simulink model "Noh_Nofusion"  (R2020b)
settings: Solver=FixedStepAuto  StartTime=0.0  StopTime=Inf  FixedStep=0.01  RelTol=1e-3
PostLoadFcn:
  | if any(exist('dsrtsu_mdlpostloadfcn', 'file') ~= 0), dsrtsu_mdlpostloadfcn('Execute', bdroot); end
InitFcn:
  | , if any(exist('rtifpga_mdlclblib', 'file') ~= 0), rtifpga_mdlclblib('Init', bdroot); end,
  | , if any(exist('dsmpb_private', 'file') ~= 0), dsmpb_private('dsmpb_mdlclblib', 'Init', bdroot); end,
undefined symbols (not defined in the file): ACC_TimeGap_DecSetSwt, ACC_TimeGap_IncSetSwt, AccelPedalPosn, AccelPedalPosnVldty, AccelPedlPosnDiagc, AccPedalOverride, ACU_ShiftInProgress, ADAS_Posn_CurLane, AESSwtReq, ALC_SwtReq, BrkPedalSts, CC_ACC_CANCEL_OFFSwt, CC_ACC_CRUISE_OFFSwt, CC_ACC_DecSetSpd_SetSwt, CC_ACC_IncSetSpd_ResuSwt, CC_ACCSwtErr, CharSpd_ms, CSA_NODE, CURRENT_GEAR, CurrentGearValid, DiscIntNeverNeededParam, DrvDoorSts, DrvSBR, DrvTrqReqOvld, ECMACCInterface, ECMRespACC, ELKSwtReq, EngLimpHomeSts, EngSpd, EngState, EngState_PHEV, EngTrqMaxActSpd, EngTrqMinAct, EPS_DrvInpTrqVal_HighReslolution, EPS_FailSts, EPS_LKATorqOvrlDlvd, EPS_LKATorqOvrlDlvdVld, EPS_LKATrqOvlDlvdSts, EPS_SteerMod, EPS_TrqSnsrSts, EQ4_APPINFO, EQ4_LA_ELEM, EQ4_LA_HDR, EQ4_LAP_ELEM, EQ4_LAP_HDR, EQ4_LH_ELEM, EQ4_LH_HDR, EQ4_LRE_ELEM, EQ4_LRE_HDR, ESS_PedSwtReq, ESS_VehSwtReq, FFogLmpSts_F_Pbox, FLWheelDriveDirection, FLWheelSpd, FrntWiprSwtSts, FrntWshrSwtSts, FRWheelDriveDirection, FRWheelSpd, HazardLmpSwtSts, HCU_AccelPedalPosn_Diag ... (+153)
libraries: simulink x132, dsmpblib x27
(part 6 of 14)

== system Noh_Nofusion/LPV/HAP_Pack ==
  In1 : Inport
  Bus Assignment2 : BusAssignment  AssignedSignals=USS_FrontSys_Status,USS_FLCNear_Obj_Confidence,USS_FLCNear_Obj_Pos_X,USS_FLCNear_Obj_Pos_Y,USS_FLMNear_Obj_Confidence,USS_FLMNear_Obj_Pos_X,USS_FLMNear_Obj_Pos_Y,USS_FRMNear_Obj_Confidence,USS_FRMNear_Obj_Pos_X,USS_FRMNear_Obj_Pos_Y,USS_FRCNear_Obj_Confidence,USS_FRCNear_Obj_Pos_X,USS_FRCNear_Obj_Pos_Y,APS_WorkSts,DVRWorkSts
  Bus Selector18 : BusSelector  OutputSignals=HAP_NODE.HAP_FD6_MSG.USS_FrontSys_Status,HAP_NODE.HAP_FD6_MSG.USS_FLCNear_Obj_Confidence,HAP_NODE.HAP_FD6_MSG.USS_FLCNear_Obj_Pos_X,HAP_NODE.HAP_FD6_MSG.USS_FLCNear_Obj_Pos_Y,HAP_NODE.HAP_FD6_MSG.USS_FLMNear_Obj_Confidence,HAP_NODE.HAP_FD6_MSG.USS_FLMNear_Obj_Pos_X,HAP_NODE.HAP_FD6_MSG.USS_FLMNear_Obj_Pos_Y,HAP_NODE.HAP_FD6_MSG.USS_FRMNear_Obj_Confidence,HAP_NODE.HAP_FD6_MSG.USS_FRMNear_Obj_Pos_X,HAP_NODE.HAP_FD6_MSG.USS_FRMNear_Obj_Pos_Y,HAP_NODE.HAP_FD6_MSG.USS_FRCNear_Obj_Confidence,HAP_NODE.HAP_FD6_MSG.USS_FRCNear_Obj_Pos_X,HAP_NODE.HAP_FD6_MSG.USS_FRCNear_Obj_Pos_Y,HAP_NODE.HAP_FD1_MSG.APS_WorkSts,HAP_NODE.HAP_FD2_MSG.DVRWorkSts
  Constant3 : Constant  Value=0  OutDataTypeStr=Bus: VCAN_HAP_MSG_BUS
  VSM_VCAN_HAP : Outport
  wires:
  Bus Assignment2/1 -> VSM_VCAN_HAP/1
  Bus Selector18/15 -> Bus Assignment2/16  "<DVRWorkSts>"
  Bus Selector18/14 -> Bus Assignment2/15  "<APS_WorkSts>"
  Bus Selector18/13 -> Bus Assignment2/14  "<USS_FRCNear_Obj_Pos_Y>"
  Bus Selector18/12 -> Bus Assignment2/13  "<USS_FRCNear_Obj_Pos_X>"
  Bus Selector18/11 -> Bus Assignment2/12  "<USS_FRCNear_Obj_Confidence>"
  Bus Selector18/10 -> Bus Assignment2/11  "<USS_FRMNear_Obj_Pos_Y>"
  Bus Selector18/9 -> Bus Assignment2/10  "<USS_FRMNear_Obj_Pos_X>"
  Bus Selector18/8 -> Bus Assignment2/9  "<USS_FRMNear_Obj_Confidence>"
  Bus Selector18/7 -> Bus Assignment2/8  "<USS_FLMNear_Obj_Pos_Y>"
  Bus Selector18/6 -> Bus Assignment2/7  "<USS_FLMNear_Obj_Pos_X>"
  Bus Selector18/5 -> Bus Assignment2/6  "<USS_FLMNear_Obj_Confidence>"
  Bus Selector18/4 -> Bus Assignment2/5  "<USS_FLCNear_Obj_Pos_Y>"
  Bus Selector18/3 -> Bus Assignment2/4  "<USS_FLCNear_Obj_Pos_X>"
  Bus Selector18/2 -> Bus Assignment2/3  "<USS_FLCNear_Obj_Confidence>"
  Bus Selector18/1 -> Bus Assignment2/2  "<USS_FrontSys_Status>"
  Constant3/1 -> Bus Assignment2/1
  In1/1 -> Bus Selector18/1

== system Noh_Nofusion/LPV/HUT_Pack ==
  In1 : Inport
  Bus Assignment1 : BusAssignment  AssignedSignals=CR_BrkgReq
  Bus Assignment2 : BusAssignment  AssignedSignals=IFC_SnvtySet,LKASwtReq,LCKSwtReq,ELKSwtReq,ESS_PedSwtReq,ESS_VehSwtReq,LDWSwtReq,TSRSwtReq,TSRWarnSwtReq,ICA_HandsOffSwtReq,ISLSwtReq,TSR_SnvtySet,LSSWarnFormSwtReq,LSSSwtReq,IntelligentEvaSwtReq,AESSwtReq,HWA_SwtReq,HWA_SnvtySet,ALC_SwtReq
  Bus Selector16 : BusSelector  OutputSignals=HUT_NODE.HUT_FD1_MSG.IFC_SnvtySet,HUT_NODE.HUT_FD1_MSG.LKASwtReq,HUT_NODE.HUT_FD1_MSG.LCKSwtReq,HUT_NODE.HUT_FD1_MSG.ELKSwtReq,HUT_NODE.HUT_FD1_MSG.ESS_PedSwtReq,HUT_NODE.HUT_FD1_MSG.ESS_VehSwtReq,HUT_NODE.HUT_FD1_MSG.LDWSwtReq,HUT_NODE.HUT_FD1_MSG.TSRSwtReq,HUT_NODE.HUT_FD1_MSG.TSRWarnSwtReq,HUT_NODE.HUT_FD1_MSG.ICA_HandsOffSwtReq,HUT_NODE.HUT_FD1_MSG.ISLSwtReq,HUT_NODE.HUT_FD1_MSG.TSR_SnvtySet,HUT_NODE.HUT_FD1_MSG.LSSWarnFormSwtReq,HUT_NODE.HUT_FD1_MSG.LSSSwtReq,HUT_NODE.HUT_FD1_MSG.IntelligentEvaSwtReq,HUT_NODE.HUT_FD1_MSG.AESSwtReq,HUT_NODE.HUT_FD1_MSG.HWA_SwtReq,HUT_NODE.HUT_FD1_MSG.HWA_SnvtySet,HUT_NODE.HUT_FD1_MSG.ALC_SwtReq,CR_NODE.CR_FD1_MSG.CR_BrkgReq
  Constant1 : Constant  Value=0  OutDataTypeStr=Bus: VCAN_CR_MSG_BUS
  Constant3 : Constant  Value=0  OutDataTypeStr=Bus: VCAN_HUT_MSG_BUS
  VSM_VCAN_HUT : Outport
  VSM_VCAN_CR : Outport  Port=2
  wires:
  Bus Assignment1/1 -> VSM_VCAN_CR/1
  Bus Selector16/20 -> Bus Assignment1/2  "<CR_BrkgReq>"
  Constant1/1 -> Bus Assignment1/1
  Bus Assignment2/1 -> VSM_VCAN_HUT/1
  Bus Selector16/19 -> Bus Assignment2/20  "<ALC_SwtReq>"
  Bus Selector16/18 -> Bus Assignment2/19  "<HWA_SnvtySet>"
  Bus Selector16/17 -> Bus Assignment2/18  "<HWA_SwtReq>"
  Bus Selector16/16 -> Bus Assignment2/17  "<AESSwtReq>"
  Bus Selector16/15 -> Bus Assignment2/16  "<IntelligentEvaSwtReq>"
  Bus Selector16/14 -> Bus Assignment2/15  "<LSSSwtReq>"
  Bus Selector16/13 -> Bus Assignment2/14  "<LSSWarnFormSwtReq>"
  Bus Selector16/12 -> Bus Assignment2/13  "<TSR_SnvtySet>"
  Bus Selector16/11 -> Bus Assignment2/12  "<ISLSwtReq>"
  Bus Selector16/10 -> Bus Assignment2/11  "<ICA_HandsOffSwtReq>"
  Bus Selector16/9 -> Bus Assignment2/10  "<TSRWarnSwtReq>"
  Bus Selector16/8 -> Bus Assignment2/9  "<TSRSwtReq>"
  Bus Selector16/7 -> Bus Assignment2/8  "<LDWSwtReq>"
  Bus Selector16/6 -> Bus Assignment2/7  "<ESS_VehSwtReq>"
  Bus Selector16/5 -> Bus Assignment2/6  "<ESS_PedSwtReq>"
  Bus Selector16/4 -> Bus Assignment2/5  "<ELKSwtReq>"
  Bus Selector16/3 -> Bus Assignment2/4  "<LCKSwtReq>"
  Bus Selector16/2 -> Bus Assignment2/3  "<LKASwtReq>"
  Bus Selector16/1 -> Bus Assignment2/2  "<IFC_SnvtySet>"
  Constant3/1 -> Bus Assignment2/1
  In1/1 -> Bus Selector16/1

== system Noh_Nofusion/LPV/Subsystem ==
  In1 : Inport
  Bus Assignment2 : BusAssignment  AssignedSignals=ACAmbTemp
  Bus Selector11 : BusSelector  OutputSignals=AC_NEDE.AC2_MSG.ACAmbTemp
  Constant3 : Constant  Value=0  OutDataTypeStr=Bus: VCAN_AC_MSG_BUS
  <ACAmbTemp> : Outport
  wires:
  Bus Assignment2/1 -> <ACAmbTemp>/1
  Constant3/1 -> Bus Assignment2/1
  Bus Selector11/1 -> Bus Assignment2/2  "<ACAmbTemp>"
  In1/1 -> Bus Selector11/1

== system Noh_Nofusion/LPV/Subsystem1 ==
  In1 : Inport
  Bus Assignment2 : BusAssignment  AssignedSignals=IP_VehSpdUnit
  Bus Selector15 : BusSelector  OutputSignals=IP_NODE.IP2_MSG.IP_VehSpdUnit
  Constant3 : Constant  Value=0  OutDataTypeStr=Bus: VCAN_IP_MSG_BUS
  <IP_VehSpdUnit> : Outport
  wires:
  Bus Assignment2/1 -> <IP_VehSpdUnit>/1
  Bus Selector15/1 -> Bus Assignment2/2  "<IP_VehSpdUnit>"
  Constant3/1 -> Bus Assignment2/1
  In1/1 -> Bus Selector15/1

== system Noh_Nofusion/LPV/Subsystem2 ==
  In1 : Inport
  Bus Assignment2 : BusAssignment  AssignedSignals=HighBeamSts_HC
  Bus Selector17 : BusSelector  OutputSignals=HC_NODE.HC1_MSG.HighBeamSts_HC
  Constant3 : Constant  Value=0  OutDataTypeStr=Bus: VCAN_HC_MSG_BUS
  <HighBeamSts_HC> : Outport
  wires:
  Bus Assignment2/1 -> <HighBeamSts_HC>/1
  Bus Selector17/1 -> Bus Assignment2/2  "<HighBeamSts_HC>"
  Constant3/1 -> Bus Assignment2/1
  In1/1 -> Bus Selector17/1

== system Noh_Nofusion/LPV/Subsystem3 ==
  In1 : Inport
  Bus Assignment2 : BusAssignment  AssignedSignals=HoodSts_F_Pbox,FFogLmpSts_F_Pbox,RFogLmpSts_R_Pbox,LowBeamSts_F_Pbox
  Bus Selector12 : BusSelector  OutputSignals=PBOX_NODE.F_PBOX1_MSG.HoodSts_F_Pbox,PBOX_NODE.F_PBOX1_MSG.FFogLmpSts_F_Pbox,PBOX_NODE.R_PBOX1_MSG.RFogLmpSts_R_Pbox,PBOX_NODE.F_PBOX1_MSG.LowBeamSts_F_Pbox
  Constant3 : Constant  Value=0  OutDataTypeStr=Bus: VCAN_PBOX_MSG_BUS
  VSM_VCAN_PBOX : Outport
  wires:
  Bus Selector12/1 -> Bus Assignment2/2  "<HoodSts_F_Pbox>"
  Bus Selector12/2 -> Bus Assignment2/3  "<FFogLmpSts_F_Pbox>"
  Bus Selector12/3 -> Bus Assignment2/4  "<RFogLmpSts_R_Pbox>"
  Bus Selector12/4 -> Bus Assignment2/5  "<LowBeamSts_F_Pbox>"
  Constant3/1 -> Bus Assignment2/1
  In1/1 -> Bus Selector12/1
  Bus Assignment2/1 -> VSM_VCAN_PBOX/1

== system Noh_Nofusion/LPV/Subsystem4 ==
  In1 : Inport
  Bus Assignment4 : BusAssignment  AssignedSignals=HCU_BrkPedalSts,HCU_AccelPedalPosn_Diag,HCU_ACCInterface,HCU_PowertrainSts,ACU_ShiftInProgress,HCU_DrvMod,HCU_PTDrvMod,DrvTrqReqOvld,HCU_GearSts
  Bus Selector11 : BusSelector  OutputSignals=HCU_NODE.HCU_FD1_MSG.HCU_BrkPedalSts,HCU_NODE.HCU_FD1_MSG.HCU_AccelPedalPosn_Diag,HCU_NODE.HCU_FD1_MSG.HCU_ACCInterface,HCU_NODE.HCU_FD1_MSG.HCU_PowertrainSts,HCU_NODE.HCU_FD1_MSG.ACU_ShiftInProgress,HCU_NODE.HCU_FD3_MSG.HCU_DrvMod,HCU_NODE.HCU_FD3_MSG.HCU_PTDrvMod,HCU_NODE.HCU_FD3_MSG.DrvTrqReqOvld,HCU_NODE.HCU_FD3_MSG.HCU_GearSts
  Constant4 : Constant  Value=0  OutDataTypeStr=Bus: VCAN_HCU_MSG_BUS
  Out1 : Outport
  wires:
  In1/1 -> Bus Selector11/1
  Bus Selector11/9 -> Bus Assignment4/10  "<HCU_GearSts>"
  Bus Selector11/7 -> Bus Assignment4/8  "<HCU_PTDrvMod>"
  Bus Selector11/3 -> Bus Assignment4/4  "<HCU_ACCInterface>"
  Bus Assignment4/1 -> Out1/1
  Bus Selector11/2 -> Bus Assignment4/3  "<HCU_AccelPedalPosn_Diag>"
  Bus Selector11/5 -> Bus Assignment4/6  "<ACU_ShiftInProgress>"
  Bus Selector11/8 -> Bus Assignment4/9  "<DrvTrqReqOvld>"
  Bus Selector11/1 -> Bus Assignment4/2  "<HCU_BrkPedalSts>"
  Constant4/1 -> Bus Assignment4/1
  Bus Selector11/6 -> Bus Assignment4/7  "<HCU_DrvMod>"
  Bus Selector11/4 -> Bus Assignment4/5  "<HCU_PowertrainSts>"

== system Noh_Nofusion/LPV/Subsystem5 ==
  TOS_P0_TARGET_LINE : Inport  OutDataTypeStr=Bus: TOS_P0_TARGET_LINE_BUS  PortDimensions=1  BusOutputAsStruct=on
  VSM_HMI : Inport  Port=2  OutDataTypeStr=Bus: VSM_HMI_BUS  PortDimensions=1  BusOutputAsStruct=on
  VSM_ReqMRC : Inport  Port=3  OutDataTypeStr=uint8
  vxvRefMs : Inport  Port=4  OutDataTypeStr=single  PortDimensions=1  BusOutputAsStruct=on
  kapTraj : Inport  Port=5  OutDataTypeStr=single  PortDimensions=1  BusOutputAsStruct=on
  PLAN_ALC_DECS : Inport  Port=6  OutDataTypeStr=Bus: PLAN_ALC_DECS_BUS  PortDimensions=1  BusOutputAsStruct=on
  RFM_ROAD : Inport  Port=7  OutDataTypeStr=Bus: RFM_ROAD_BUS  PortDimensions=1  BusOutputAsStruct=on
  RFM_UpdateCnt : Inport  Port=8  OutDataTypeStr=uint32  PortDimensions=1  BusOutputAsStruct=on
  RFM_BRANCH_LANE : Inport  Port=9  OutDataTypeStr=Bus: RFM_LANE_BUS  PortDimensions=1  BusOutputAsStruct=on
  RFM_LEFT_LANE : Inport  Port=10  OutDataTypeStr=Bus: RFM_LANE_BUS  PortDimensions=1  BusOutputAsStruct=on
  RFM_CURRENT_LANE : Inport  Port=11  OutDataTypeStr=Bus: RFM_LANE_BUS  PortDimensions=1  BusOutputAsStruct=on
  RFM_RIGHT_LANE : Inport  Port=12  OutDataTypeStr=Bus: RFM_LANE_BUS  PortDimensions=1  BusOutputAsStruct=on
  RFM_INTERSEC_ALERT : Inport  Port=13  OutDataTypeStr=Bus: RFM_INTERSEC_ALERT_BUS  PortDimensions=1  BusOutputAsStruct=on
  RFM_BRANCH : Inport  Port=14  OutDataTypeStr=Bus: RFM_BRANCH_BUS  PortDimensions=1  BusOutputAsStruct=on
  RFM_REC_LANES : Inport  Port=15  OutDataTypeStr=Bus: RFM_REC_LANES_BUS  PortDimensions=1  BusOutputAsStruct=on
  RFM_LINE_L1 : Inport  Port=16  OutDataTypeStr=Bus: RFM_LINE_BUS  PortDimensions=1  BusOutputAsStruct=on
  RFM_LINE_R1 : Inport  Port=17  OutDataTypeStr=Bus: RFM_LINE_BUS  PortDimensions=1  BusOutputAsStruct=on
  RFM_LINE_L2 : Inport  Port=18  OutDataTypeStr=Bus: RFM_LINE_BUS  PortDimensions=1  BusOutputAsStruct=on
  RFM_LINE_R2 : Inport  Port=19  OutDataTypeStr=Bus: RFM_LINE_BUS  PortDimensions=1  BusOutputAsStruct=on
  RFM_LINE_L3 : Inport  Port=20  OutDataTypeStr=Bus: RFM_LINE_BUS  PortDimensions=1  BusOutputAsStruct=on
  RFM_LINE_R3 : Inport  Port=21  OutDataTypeStr=Bus: RFM_LINE_BUS  PortDimensions=1  BusOutputAsStruct=on
  RFM_LINE_CL : Inport  Port=22  OutDataTypeStr=Bus: RFM_LINE_BUS  PortDimensions=1  BusOutputAsStruct=on
  RFM_LINE_LB : Inport  Port=23  OutDataTypeStr=Bus: RFM_LINE_BUS  PortDimensions=1  BusOutputAsStruct=on
  RFM_LINE_RB : Inport  Port=24  OutDataTypeStr=Bus: RFM_LINE_BUS  PortDimensions=1  BusOutputAsStruct=on
  RFM_LINE_PRED : Inport  Port=25  OutDataTypeStr=Bus: RFM_LINE_BUS  PortDimensions=1  BusOutputAsStruct=on
  RFM_LINEF_LB : Inport  Port=26  OutDataTypeStr=Bus: RFM_LINE_BUS  PortDimensions=1  BusOutputAsStruct=on
  RFM_LINEF_RB : Inport  Port=27  OutDataTypeStr=Bus: RFM_LINE_BUS  PortDimensions=1  BusOutputAsStruct=on
  RFM_LINE_ENTRY_CL : Inport  Port=28  OutDataTypeStr=Bus: RFM_LINE_BUS  PortDimensions=1  BusOutputAsStruct=on
  RFM_LINE_EXIT_CL : Inport  Port=29  OutDataTypeStr=Bus: RFM_LINE_BUS  PortDimensions=1  BusOutputAsStruct=on
  EQ4_LH_HDR : Inport  Port=30  OutDataTypeStr=Bus: EQ4_LH_HDR_BUS  PortDimensions=1  BusOutputAsStruct=on
  EQ4_LH_ELEM : Inport  Port=31  OutDataTypeStr=Bus: EQ4_LH_ELEM_BUS  PortDimensions=1  BusOutputAsStruct=on
  EQ4_LH_ELEM1 : Inport  Port=32  OutDataTypeStr=Bus: EQ4_LH_ELEM_BUS  PortDimensions=1  BusOutputAsStruct=on
  EQ4_LA_HDR : Inport  Port=33  OutDataTypeStr=Bus: EQ4_LA_HDR_BUS  PortDimensions=1  BusOutputAsStruct=on
  EQ4_LA_ELEM : Inport  Port=34  OutDataTypeStr=Bus: EQ4_LA_ELEM_BUS  PortDimensions=1  BusOutputAsStruct=on
  EQ4_LA_ELEM1 : Inport  Port=35  OutDataTypeStr=Bus: EQ4_LA_ELEM_BUS  PortDimensions=1  BusOutputAsStruct=on
  EQ4_LA_ELEM2 : Inport  Port=36  OutDataTypeStr=Bus: EQ4_LA_ELEM_BUS  PortDimensions=1  BusOutputAsStruct=on
  EQ4_LA_ELEM3 : Inport  Port=37  OutDataTypeStr=Bus: EQ4_LA_ELEM_BUS  PortDimensions=1  BusOutputAsStruct=on
  EQ4_LRE_HDR : Inport  Port=38  OutDataTypeStr=Bus: EQ4_LRE_HDR_BUS  PortDimensions=1  BusOutputAsStruct=on
  EQ4_LRE_ELEM : Inport  Port=39  OutDataTypeStr=Bus: EQ4_LRE_ELEM_BUS  PortDimensions=1  BusOutputAsStruct=on
  EQ4_LRE_ELEM1 : Inport  Port=40  OutDataTypeStr=Bus: EQ4_LRE_ELEM_BUS  PortDimensions=1  BusOutputAsStruct=on
  RFM_TSR : Inport  Port=41  OutDataTypeStr=Bus: RFM_TSR_BUS  PortDimensions=1  BusOutputAsStruct=on
  Bus Assignment1 : BusAssignment  AssignedSignals=EQ4_LH_HDR,EQ4_LH_ELEM
  Bus Assignment2 : BusAssignment  AssignedSignals=EQ4_LRE_HDR,EQ4_LRE_ELEM
  Bus Assignment3 : BusAssignment  AssignedSignals=EQ4_LA_HDR,EQ4_LA_ELEM
  Constant1 : Constant  Value=0  OutDataTypeStr=Bus: EQ4_LA_BUS
  Constant2 : Constant  Value=0  OutDataTypeStr=Bus: EQ4_LH_BUS
  Constant3 : Constant  Value=0  OutDataTypeStr=Bus: EQ4_LRE_BUS
  For Each Subsystem1 : Subsystem  TreatAsAtomicUnit=on
  For Each Subsystem2 : Subsystem  TreatAsAtomicUnit=on
  For Each Subsystem3 : Subsystem  TreatAsAtomicUnit=on
  LSM : ModelReference  ModelNameDialog=PubIfDecisionLSM_MDL.slx  SimulationMode=Normal  ModelReferenceVersion=1.510
  Matrix Concatenate : Concatenate  Mode=Multidimensional array
  Matrix Concatenate1 : Concatenate  NumInputs=4  Mode=Multidimensional array
  Matrix Concatenate2 : Concatenate  Mode=Multidimensional array
  Terminator : Terminator
  LSM_TJA_ICA : Outport  OutDataTypeStr=Bus: LSM_TJA_ICA_BUS  PortDimensions=1  BusOutputAsStruct=on
  LSM_LCK : Outport  Port=2  OutDataTypeStr=Bus: LSM_LCK_BUS  PortDimensions=1  BusOutputAsStruct=on
  LSM_HWA : Outport  Port=3  OutDataTypeStr=Bus: LSM_HWA_BUS  PortDimensions=1  BusOutputAsStruct=on
  LSM_ESS : Outport  Port=4  OutDataTypeStr=Bus: LSM_ESS_BUS  PortDimensions=1  BusOutputAsStruct=on
  LSM_UpdateCnt : Outport  Port=5  OutDataTypeStr=uint32  PortDimensions=1  BusOutputAsStruct=on
  LSM_PilotTurnSwSts : Outport  Port=6  OutDataTypeStr=uint8  PortDimensions=1  BusOutputAsStruct=on
  LSM_PilotSts : Outport  Port=7  OutDataTypeStr=uint8  PortDimensions=1  BusOutputAsStruct=on
  LSM_PilotNohExitDist : Outport  Port=8  OutDataTypeStr=uint16  PortDimensions=1  BusOutputAsStruct=on
  LSM_PilotSPLDist : Outport  Port=9  OutDataTypeStr=uint16  PortDimensions=1  BusOutputAsStruct=on
  LSM_PilotSPL : Outport  Port=10  OutDataTypeStr=uint8  PortDimensions=1  BusOutputAsStruct=on
  LSM_PilotRoadSts : Outport  Port=11  OutDataTypeStr=uint8  PortDimensions=1  BusOutputAsStruct=on
  wires:
  VSM_ReqMRC/1 -> Terminator/1
  RFM_TSR/1 -> LSM/33
  RFM_LINE_EXIT_CL/1 -> LSM/32
  RFM_LINE_ENTRY_CL/1 -> LSM/31
  RFM_LINEF_RB/1 -> LSM/30
  RFM_LINEF_LB/1 -> LSM/29
  RFM_LINE_PRED/1 -> LSM/28
  RFM_LINE_RB/1 -> LSM/27
  RFM_LINE_LB/1 -> LSM/26
  RFM_LINE_CL/1 -> LSM/25
  RFM_LINE_R3/1 -> LSM/24
  RFM_LINE_L3/1 -> LSM/23
  RFM_LINE_R2/1 -> LSM/22
  RFM_LINE_L2/1 -> LSM/21
  RFM_LINE_R1/1 -> LSM/20
  RFM_LINE_L1/1 -> LSM/19
  RFM_REC_LANES/1 -> LSM/18
  RFM_BRANCH/1 -> LSM/17
  RFM_INTERSEC_ALERT/1 -> LSM/16
  RFM_RIGHT_LANE/1 -> LSM/15
  RFM_CURRENT_LANE/1 -> LSM/14
  RFM_LEFT_LANE/1 -> LSM/13
  RFM_BRANCH_LANE/1 -> LSM/12
  RFM_UpdateCnt/1 -> LSM/11
  RFM_ROAD/1 -> LSM/10
  PLAN_ALC_DECS/1 -> LSM/9
  kapTraj/1 -> LSM/8
  vxvRefMs/1 -> LSM/7
  LSM/10 -> LSM_PilotSPL/1
  EQ4_LA_HDR/1 -> Bus Assignment3/2
  Matrix Concatenate1/1 -> For Each Subsystem3/1(In1)
  EQ4_LA_ELEM/1 -> Matrix Concatenate1/1
  EQ4_LRE_ELEM/1 -> Matrix Concatenate2/1
  EQ4_LA_ELEM3/1 -> Matrix Concatenate1/4
  Constant2/1 -> Bus Assignment1/1
  Constant1/1 -> Bus Assignment3/1
  EQ4_LH_ELEM/1 -> Matrix Concatenate/1
  Bus Assignment1/1 -> LSM/2
  LSM/6 -> LSM_PilotTurnSwSts/1
  LSM/2 -> LSM_LCK/1
  VSM_HMI/1 -> LSM/6
  Matrix Concatenate2/1 -> For Each Subsystem2/1(In1)
  LSM/7 -> LSM_PilotSts/1
  EQ4_LRE_ELEM1/1 -> Matrix Concatenate2/2
  TOS_P0_TARGET_LINE/1 -> LSM/5
  EQ4_LRE_HDR/1 -> Bus Assignment2/2
  Bus Assignment3/1 -> LSM/3
  LSM/4 -> LSM_ESS/1
  EQ4_LA_ELEM2/1 -> Matrix Concatenate1/3
  EQ4_LH_ELEM1/1 -> Matrix Concatenate/2
  LSM/9 -> LSM_PilotSPLDist/1
  LSM/3 -> LSM_HWA/1
  Bus Assignment2/1 -> LSM/4
  LSM/8 -> LSM_PilotNohExitDist/1
  LSM/11 -> LSM_PilotRoadSts/1
  LSM/1 -> LSM_TJA_ICA/1
  For Each Subsystem3/1(Out1) -> Bus Assignment3/3
  Constant3/1 -> Bus Assignment2/1
  EQ4_LA_ELEM1/1 -> Matrix Concatenate1/2
  Matrix Concatenate/1 -> For Each Subsystem1/1(In1)
  EQ4_LH_HDR/1 -> Bus Assignment1/2
  LSM/5 -> LSM_UpdateCnt/1
  For Each Subsystem2/1(Out1) -> Bus Assignment2/3
  For Each Subsystem1/1(Out1) -> Bus Assignment1/3

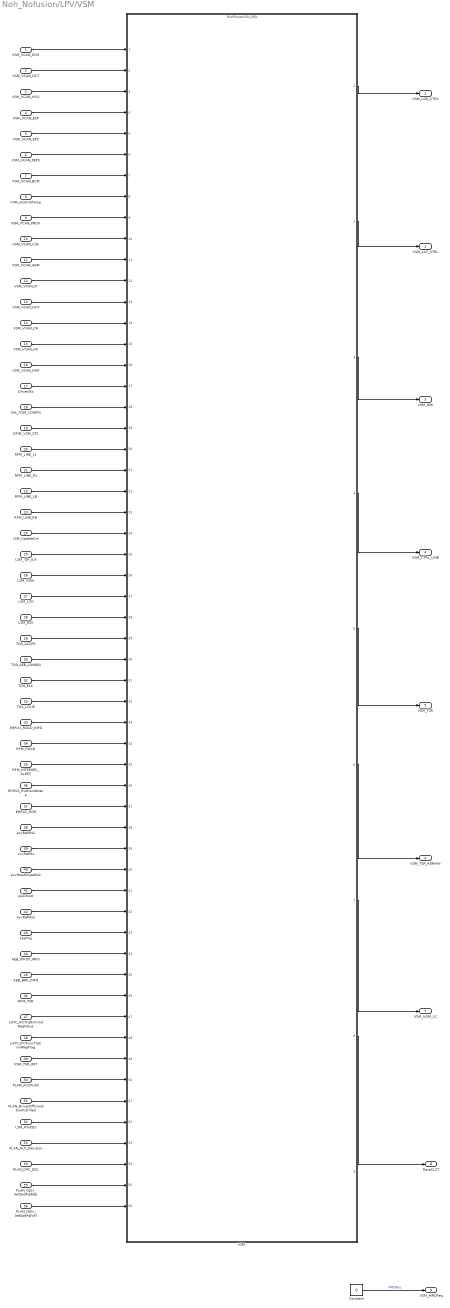
== system Noh_Nofusion/LPV/VSM ==
  VSM_VCAN_ECM : Inport  OutDataTypeStr=Bus: VCAN_ECM_MSG_BUS  PortDimensions=1  BusOutputAsStruct=on
  VSM_VCAN_DCT : Inport  Port=2  OutDataTypeStr=Bus: VCAN_DCT_MSG_BUS  PortDimensions=1  BusOutputAsStruct=on
  VSM_VCAN_HCU : Inport  Port=3  OutDataTypeStr=Bus: VCAN_HCU_MSG_BUS  PortDimensions=1  BusOutputAsStruct=on
  VSM_VCAN_ESP : Inport  Port=4  OutDataTypeStr=Bus: VCAN_ESP_MSG_BUS  PortDimensions=1  BusOutputAsStruct=on
  VSM_VCAN_EPS : Inport  Port=5  OutDataTypeStr=Bus: VCAN_EPS_MSG_BUS  PortDimensions=1  BusOutputAsStruct=on
  VSM_VCAN_PEPS : Inport  Port=6  OutDataTypeStr=Bus: VCAN_PEPS_MSG_BUS  PortDimensions=1  BusOutputAsStruct=on
  VSM_VCAN_BCM : Inport  Port=7  OutDataTypeStr=Bus: VCAN_BCM_MSG_BUS  PortDimensions=1  BusOutputAsStruct=on
  VSM_ACAmbTemp : Inport  Port=8  OutDataTypeStr=Bus: VCAN_AC_MSG_BUS  PortDimensions=1  BusOutputAsStruct=on
  VSM_VCAN_PBOX : Inport  Port=9  OutDataTypeStr=Bus: VCAN_PBOX_MSG_BUS  PortDimensions=1  BusOutputAsStruct=on
  VSM_VCAN_CSA : Inport  Port=10  OutDataTypeStr=Bus: VCAN_CSA_MSG_BUS  PortDimensions=1  BusOutputAsStruct=on
  VSM_VCAN_ABM : Inport  Port=11  OutDataTypeStr=Bus: VCAN_ABM_MSG_BUS  PortDimensions=1  BusOutputAsStruct=on
  VSM_VCAN_IP : Inport  Port=12  OutDataTypeStr=Bus: VCAN_IP_MSG_BUS  PortDimensions=1  BusOutputAsStruct=on
  VSM_VCAN_HUT : Inport  Port=13  OutDataTypeStr=Bus: VCAN_HUT_MSG_BUS  PortDimensions=1  BusOutputAsStruct=on
  VSM_VCAN_CR : Inport  Port=14  OutDataTypeStr=Bus: VCAN_CR_MSG_BUS  PortDimensions=1  BusOutputAsStruct=on
  VSM_VCAN_HC : Inport  Port=15  OutDataTypeStr=Bus: VCAN_HC_MSG_BUS  PortDimensions=1  BusOutputAsStruct=on
  VSM_VCAN_HAP : Inport  Port=16  OutDataTypeStr=Bus: VCAN_HAP_MSG_BUS  PortDimensions=1  BusOutputAsStruct=on
  DriverSts : Inport  Port=17  OutDataTypeStr=uint8  PortDimensions=1  BusOutputAsStruct=on
  CAL_VSM_CONFIG : Inport  Port=18  OutDataTypeStr=Bus: CAL_VSM_CONFIG_BUS  PortDimensions=1  BusOutputAsStruct=on
  DFIM_VSM_STS : Inport  Port=19  OutDataTypeStr=Bus: DFIM_VSM_STS_BUS  PortDimensions=1  BusOutputAsStruct=on
  RFM_LINE_L1 : Inport  Port=20  OutDataTypeStr=Bus: RFM_LINE_BUS  PortDimensions=1  BusOutputAsStruct=on
  RFM_LINE_R1 : Inport  Port=21  OutDataTypeStr=Bus: RFM_LINE_BUS  PortDimensions=1  BusOutputAsStruct=on
  RFM_LINE_LB : Inport  Port=22  OutDataTypeStr=Bus: RFM_LINE_BUS  PortDimensions=1  BusOutputAsStruct=on
  RFM_LINE_RB : Inport  Port=23  OutDataTypeStr=Bus: RFM_LINE_BUS  PortDimensions=1  BusOutputAsStruct=on
  LSM_UpdateCnt : Inport  Port=24  OutDataTypeStr=uint32  PortDimensions=1  BusOutputAsStruct=on
  LSM_TJA_ICA : Inport  Port=25  OutDataTypeStr=Bus: LSM_TJA_ICA_BUS  PortDimensions=1  BusOutputAsStruct=on
  LSM_HWA : Inport  Port=26  OutDataTypeStr=Bus: LSM_HWA_BUS  PortDimensions=1  BusOutputAsStruct=on
  LSM_LCK : Inport  Port=27  OutDataTypeStr=Bus: LSM_LCK_BUS  PortDimensions=1  BusOutputAsStruct=on
  LSM_ESS : Inport  Port=28  OutDataTypeStr=Bus: LSM_ESS_BUS  PortDimensions=1  BusOutputAsStruct=on
  TOS_ACCP0 : Inport  Port=29  OutDataTypeStr=Bus: TOS_ACCP0_BUS  PortDimensions=1  BusOutputAsStruct=on
  TOS_AEB_LONOBJ : Inport  Port=30  OutDataTypeStr=Bus: TOS_AEB_LONOBJ_BUS  PortDimensions=1  BusOutputAsStruct=on
  TOS_ELK : Inport  Port=31  OutDataTypeStr=Bus: TOS_ELK_BUS  PortDimensions=1  BusOutputAsStruct=on
  TOS_LCKIE : Inport  Port=32  OutDataTypeStr=Bus: TOS_LCKIE_BUS  PortDimensions=1  BusOutputAsStruct=on
  EHRV2_ROAD_INFO : Inport  Port=33  OutDataTypeStr=Bus: EHRV2_ROAD_INFO_BUS  PortDimensions=1  BusOutputAsStruct=on
  RFM_ROAD : Inport  Port=34  OutDataTypeStr=Bus: RFM_ROAD_BUS  PortDimensions=1  BusOutputAsStruct=on
  RFM_INTERSEC_ALERT : Inport  Port=35  OutDataTypeStr=Bus: RFM_INTERSEC_ALERT_BUS  PortDimensions=1  BusOutputAsStruct=on
  EHRV2_HutHandshake : Inport  Port=36  OutDataTypeStr=uint8  PortDimensions=1  BusOutputAsStruct=on
  EHRV2_HDR : Inport  Port=37  OutDataTypeStr=Bus: EHRV2_HDR_BUS  PortDimensions=1  BusOutputAsStruct=on
  axvRefMs2 : Inport  Port=38  OutDataTypeStr=single  PortDimensions=1  BusOutputAsStruct=on
  vxvRefMs : Inport  Port=39  OutDataTypeStr=single  PortDimensions=1  BusOutputAsStruct=on
  axvRoadSlopeMs2 : Inport  Port=40  OutDataTypeStr=single  PortDimensions=1  BusOutputAsStruct=on
  psiDtOpt : Inport  Port=41  OutDataTypeStr=single  PortDimensions=1  BusOutputAsStruct=on
  ayvRefMs2 : Inport  Port=42  OutDataTypeStr=single  PortDimensions=1  BusOutputAsStruct=on
  kapTraj : Inport  Port=43  OutDataTypeStr=single  PortDimensions=1  BusOutputAsStruct=on
  AEB_IPHUT_INFO : Inport  Port=44  OutDataTypeStr=Bus: AEB_IPHUT_INFO_BUS  PortDimensions=1  BusOutputAsStruct=on
  AEB_BRK_INFO : Inport  Port=45  OutDataTypeStr=Bus: AEB_BRK_INFO_BUS  PortDimensions=1  BusOutputAsStruct=on
  RFM_TSR : Inport  Port=46  OutDataTypeStr=Bus: RFM_TSR_BUS  PortDimensions=1  BusOutputAsStruct=on
  LATC_IFCTrqOvlCmdReqValue : Inport  Port=47  OutDataTypeStr=single  PortDimensions=1  BusOutputAsStruct=on
  LATC_IFCFuncTrqCmdReqFlag : Inport  Port=48  OutDataTypeStr=uint8  PortDimensions=1  BusOutputAsStruct=on
  VSM_TSR_INIT : Inport  Port=49  OutDataTypeStr=Bus: VSM_TSR_INIT_BUS  PortDimensions=1  BusOutputAsStruct=on
  PLAN_ACCPLAN : Inport  Port=50  OutDataTypeStr=Bus: PLAN_ACCPLAN_BUS  PortDimensions=1  BusOutputAsStruct=on
  PLAN_DriverOffConditionFulfilled : Inport  Port=51  OutDataTypeStr=boolean  PortDimensions=1  BusOutputAsStruct=on
  LSM_PilotSts : Inport  Port=52  OutDataTypeStr=uint8  PortDimensions=1  BusOutputAsStruct=on
  PLAN_ALC_Decision : Inport  Port=53  OutDataTypeStr=Bus: PLAN_ALC_DECS_BUS
  PLAN_DPC_ESS : Inport  Port=54  OutDataTypeStr=Bus: PLAN_DPC_ESS_BUS
  PLAN_NOH_SetSpdAdjReq : Inport  Port=55  OutDataTypeStr=boolean
  PLAN_NOH_SetSpdAdjVal : Inport  Port=56  OutDataTypeStr=uint8
  Constant : Constant  Value=0  OutDataTypeStr=uint8
  VSM : ModelReference  ModelNameDialog=PubIfStateVSM_MDL.slx  SimulationMode=Normal  ModelReferenceVersion=1.109
  VSM_LON_CTRL : Outport  OutDataTypeStr=Bus: VSM_LON_CTRL_BUS  PortDimensions=1  BusOutputAsStruct=on
  VSM_LAT_CTRL : Outport  Port=2  OutDataTypeStr=Bus: VSM_LAT_CTRL_BUS  BusOutputAsStruct=on
  VSM_HMI : Outport  Port=3  OutDataTypeStr=Bus: VSM_HMI_BUS  PortDimensions=1  BusOutputAsStruct=on
  VSM_CTRL_LINE : Outport  Port=4  OutDataTypeStr=Bus: VSM_CTRL_LINE_BUS  PortDimensions=1  BusOutputAsStruct=on
  VSM_TSR : Outport  Port=5  OutDataTypeStr=Bus: VSM_TSR_BUS  PortDimensions=1  BusOutputAsStruct=on
  VSM_TSR_REMAIN : Outport  Port=6  OutDataTypeStr=Bus: VSM_TSR_REMAIN_BUS  BusOutputAsStruct=on
  VSM_UOM_LC : Outport  Port=7  OutDataTypeStr=Bus: VSM_UOM_LC_BUS
  DataCLCT : Outport  Port=8
  VSM_MRCReq : Outport  Port=9  OutDataTypeStr=uint8
  wires:
  Constant/1 -> VSM_MRCReq/1  "MRCReq"
  PLAN_NOH_SetSpdAdjVal/1 -> VSM/56
  PLAN_NOH_SetSpdAdjReq/1 -> VSM/55
  PLAN_DPC_ESS/1 -> VSM/54
  PLAN_ALC_Decision/1 -> VSM/53
  LSM_PilotSts/1 -> VSM/52
  PLAN_DriverOffConditionFulfilled/1 -> VSM/51
  PLAN_ACCPLAN/1 -> VSM/50
  VSM_TSR_INIT/1 -> VSM/49
  LATC_IFCFuncTrqCmdReqFlag/1 -> VSM/48
  LATC_IFCTrqOvlCmdReqValue/1 -> VSM/47
  RFM_TSR/1 -> VSM/46
  AEB_BRK_INFO/1 -> VSM/45
  AEB_IPHUT_INFO/1 -> VSM/44
  kapTraj/1 -> VSM/43
  ayvRefMs2/1 -> VSM/42
  psiDtOpt/1 -> VSM/41
  axvRoadSlopeMs2/1 -> VSM/40
  vxvRefMs/1 -> VSM/39
  axvRefMs2/1 -> VSM/38
  EHRV2_HDR/1 -> VSM/37
  EHRV2_HutHandshake/1 -> VSM/36
  RFM_INTERSEC_ALERT/1 -> VSM/35
  RFM_ROAD/1 -> VSM/34
  EHRV2_ROAD_INFO/1 -> VSM/33
  TOS_LCKIE/1 -> VSM/32
  TOS_ELK/1 -> VSM/31
  TOS_AEB_LONOBJ/1 -> VSM/30
  TOS_ACCP0/1 -> VSM/29
  LSM_ESS/1 -> VSM/28
  LSM_LCK/1 -> VSM/27
  LSM_HWA/1 -> VSM/26
  LSM_TJA_ICA/1 -> VSM/25
  LSM_UpdateCnt/1 -> VSM/24
  RFM_LINE_RB/1 -> VSM/23
  RFM_LINE_LB/1 -> VSM/22
  RFM_LINE_R1/1 -> VSM/21
  RFM_LINE_L1/1 -> VSM/20
  DFIM_VSM_STS/1 -> VSM/19
  CAL_VSM_CONFIG/1 -> VSM/18
  DriverSts/1 -> VSM/17
  VSM_VCAN_HAP/1 -> VSM/16
  VSM_VCAN_HC/1 -> VSM/15
  VSM_VCAN_CR/1 -> VSM/14
  VSM_VCAN_HUT/1 -> VSM/13
  VSM_VCAN_IP/1 -> VSM/12
  VSM_VCAN_ABM/1 -> VSM/11
  VSM_VCAN_CSA/1 -> VSM/10
  VSM_VCAN_PBOX/1 -> VSM/9
  VSM_ACAmbTemp/1 -> VSM/8
  VSM_VCAN_BCM/1 -> VSM/7
  VSM_VCAN_PEPS/1 -> VSM/6
  VSM_VCAN_EPS/1 -> VSM/5
  VSM_VCAN_ESP/1 -> VSM/4
  VSM_VCAN_HCU/1 -> VSM/3
  VSM_VCAN_DCT/1 -> VSM/2
  VSM_VCAN_ECM/1 -> VSM/1
  VSM/7 -> VSM_UOM_LC/1
  VSM/8 -> DataCLCT/1
  VSM/3 -> VSM_HMI/1
  VSM/5 -> VSM_TSR/1
  VSM/4 -> VSM_CTRL_LINE/1
  VSM/2 -> VSM_LAT_CTRL/1
  VSM/1 -> VSM_LON_CTRL/1
  VSM/6 -> VSM_TSR_REMAIN/1

== system Noh_Nofusion/SimBCM/CSALampCtrlSim ==
  SteerWheelAng : Inport
  SteerWheelAngSign : Inport  Port=2
  LeLmp : Inport  Port=3
  RiLmp : Inport  Port=4
  IDC_L2_LampReq : Inport  Port=5
  AND : Logic  AllPortsSameDT=off  OutDataTypeStr=boolean
  Chart1 : Stateflow chart  TreatAsAtomicUnit=on
      settings: PortSchema="{\"entries\":[{\"content\":{\"sides\":[{\"content\":{\"connectorIds\":[\"In2\",\"In3\",\"In1\",\"In5\",\"In4\"]},\"type\":\"ConnectorPlacement.EquallySpacedRectSide\",\"uuid\":\"39a1b1a6-dbff-4545-9b5d-a590c8e27162\"},{\"content\":{\"connectorIds\":[\"Out1\"],\"side\":\"RIGHT\"},\"type\":\"ConnectorPlacement.EquallySpacedRectSide\",\"uuid\":\"07a8f021-0c33-4101-a96c-68b7faf2bb11\"},{\"content\":{\"connectorIds\":[],\"side\":\"TOP\"},\"type\":\"ConnectorPlacement.EquallySpacedRectSide\",\"uuid\":\"7e2d5075-bd26-480f-8577-c5b818a20656\"},{\"content\":{\"connectorIds\":[],\"side\":\"HIDDEN\"},\"type\":\"ConnectorPlacement.EquallySpacedRectSide\",\"uuid\":\"ac2c995e-c314-428d-9a21-32a9c673df3a\"}]},\"type\":\"ConnectorPlacement.EquallySpacedConnector\",\"uuid\":\"d3e0c913-8ba7-48f6-b6d2-3cb01edd4105\"}],\"packageUris\":[\"http://schema.mathworks.com/mf0/Connector/R2020b\"],\"version\":\"1.0\"}"
  Chart2 : Stateflow chart  TreatAsAtomicUnit=on
      settings: PortSchema="{\"entries\":[{\"content\":{\"sides\":[{\"content\":{\"connectorIds\":[\"In2\",\"In3\",\"In1\",\"In5\",\"In4\"]},\"type\":\"ConnectorPlacement.EquallySpacedRectSide\",\"uuid\":\"39a1b1a6-dbff-4545-9b5d-a590c8e27162\"},{\"content\":{\"connectorIds\":[\"Out1\"],\"side\":\"RIGHT\"},\"type\":\"ConnectorPlacement.EquallySpacedRectSide\",\"uuid\":\"07a8f021-0c33-4101-a96c-68b7faf2bb11\"},{\"content\":{\"connectorIds\":[],\"side\":\"TOP\"},\"type\":\"ConnectorPlacement.EquallySpacedRectSide\",\"uuid\":\"7e2d5075-bd26-480f-8577-c5b818a20656\"},{\"content\":{\"connectorIds\":[],\"side\":\"HIDDEN\"},\"type\":\"ConnectorPlacement.EquallySpacedRectSide\",\"uuid\":\"ac2c995e-c314-428d-9a21-32a9c673df3a\"}]},\"type\":\"ConnectorPlacement.EquallySpacedConnector\",\"uuid\":\"d3e0c913-8ba7-48f6-b6d2-3cb01edd4105\"}],\"packageUris\":[\"http://schema.mathworks.com/mf0/Connector/R2020b\"],\"version\":\"1.0\"}"
  Compare To Constant : simulink/Logic and Bit Operations/Compare To Constant  relop===  const=3.0  OutDataTypeStr=boolean
  Compare To Constant1 : simulink/Logic and Bit Operations/Compare To Constant  relop=~=  const=3.0  OutDataTypeStr=boolean
  Constant : Constant  Value=40
  Constant2 : Constant  Value=10
  Counter1 : Subsystem
  Counter4 : Subsystem
  OR : Logic  Operator=OR  AllPortsSameDT=off  OutDataTypeStr=boolean
  OR1 : Logic  Operator=OR  AllPortsSameDT=off  OutDataTypeStr=boolean
  OR2 : Logic  Operator=OR  Inputs=4  AllPortsSameDT=off  OutDataTypeStr=boolean
  OR3 : Logic  Operator=OR  Inputs=4  AllPortsSameDT=off  OutDataTypeStr=boolean
  Product : Product
  Unit Delay : UnitDelay  SampleTime=-1  HasFrameUpgradeWarning=on
  LTurnLmpSwtSts : Outport
  RTurnLmpSwtSts : Outport  Port=2
  wires:
  Compare To Constant1/1 -> AND/1
  Unit Delay/1 -> Compare To Constant1/1
  AND/1 -> OR3/4, OR2/4
  Compare To Constant/1 -> AND/2
  IDC_L2_LampReq/1 -> Unit Delay/1, Compare To Constant/1
  RiLmp/1 -> Counter1/1(Trigger)
  Counter4/1(Short) -> OR3/2, OR/1, OR2/1
  LeLmp/1 -> Counter4/1(Trigger)
  Constant2/1 -> Chart2/4(P_LmpCloseAngClose), Chart1/4(P_LmpCloseAngClose)
  Constant/1 -> Chart1/5(P_LmpCloseAngReady), Chart2/5(P_LmpCloseAngReady)
  OR3/1 -> Chart2/1(OFF)
  OR2/1 -> Chart1/1(OFF)
  Product/1 -> Chart2/3(SteerWheelAng), Chart1/3(SteerWheelAng)
  Chart2/1(SwtSts) -> OR1/2
  Chart1/1(SwtSts) -> OR/2
  SteerWheelAngSign/1 -> Product/2  "SteerWheelAngSign"
  SteerWheelAng/1 -> Product/1  "SteerWheelAng"
  Counter1/2(Long) -> OR2/2, Chart2/2(ON)
  Counter1/1(Short) -> OR2/3, OR3/1, OR1/1
  OR/1 -> LTurnLmpSwtSts/1
  Counter4/2(Long) -> OR3/3, Chart1/2(ON)
  OR1/1 -> RTurnLmpSwtSts/1

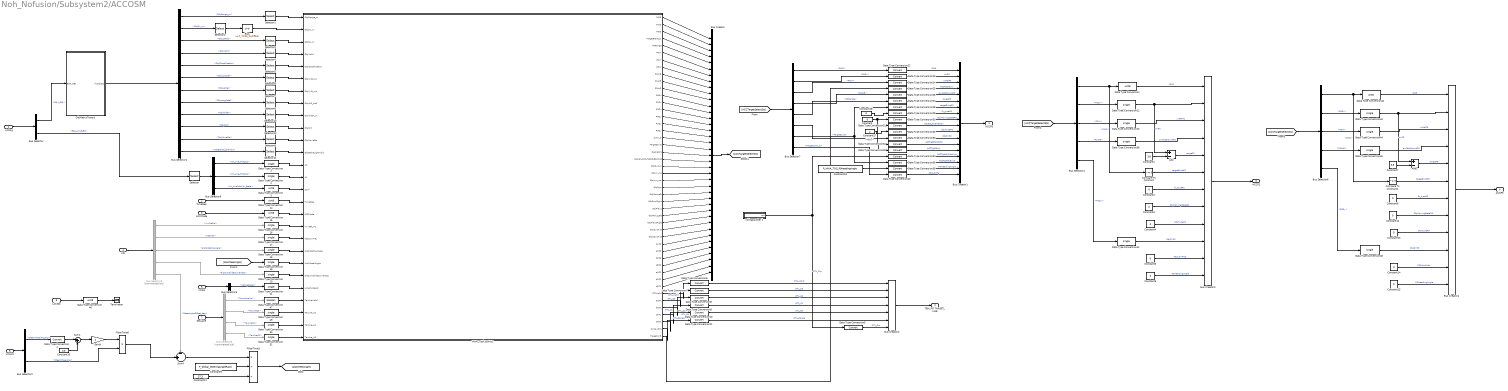
== system Noh_Nofusion/Subsystem2/ACCOSM ==
  visMsg : Inport
  TimeGap : Inport  Port=2
  ACCMode : Inport  Port=3
  VIE : Inport  Port=4
  VCAN : Inport  Port=5
  LCKSts : Inport  Port=6
  desLane : Inport  Port=7
  Add : Sum  Inputs=+-
  Add1 : Sum  Inputs=+-
  Bias : Bias  Bias=P_TOSS_DxOffset
  Bus Creator : BusCreator  Inputs=39
  Bus Creator1 : BusCreator  Inputs=18  OutDataTypeStr=Bus: TOS_ACCP0_BUS  NonVirtualBus=on
  Bus Creator2 : BusCreator  Inputs=7  OutDataTypeStr=Bus: TOS_P0_TARGET_LINE_BUS  NonVirtualBus=on
  Bus Creator3 : BusCreator  Inputs=12  OutDataTypeStr=Bus: TOS_ACCP2_BUS  NonVirtualBus=on
  Bus Creator4 : BusCreator  Inputs=12  OutDataTypeStr=Bus: TOS_ACCP3_BUS  NonVirtualBus=on
  Bus Selector : BusSelector  OutputSignals=EQ4_OBJ,EQ4_LH.EQ4_LH_ELEM
  Bus Selector4 : BusSelector  OutputSignals=P2ID,P2Dx,P2Vr,P2ArG,P2Dy
  Bus Selector6 : BusSelector  OutputSignals=P3ID,P3Dx,P3Vr,P3ArG,P3Dy
  Bus Selector7 : BusSelector  OutputSignals=P0ID,P0Dx,P0Vr,P0ArG,P0Range,P0Dy,TargetExist,TargetCutIn_b
  Bus Selector9 : BusSelector  OutputSignals=LH_Line_First_C2,LH_Line_First_C1,LH_Availability_State
  Bus Selector1 : BusSelector  OutputSignals=ObjRange_m,ObjDx_m,ObjLatPos,ObjValid,ObjClassification,ObjLongVel,ObjLatVel,ObjLongAccel,ObjWidth,ObjCnt,ObjMoveSts,ObjBrakeLightIndic
  Bus Selector2 : BusSelector  OutputSignals=CSA_NODE.CSA2_MSG.SteerWheelAngSign,CSA_NODE.CSA2_MSG.SteerWheelAng
  Bus Selector3 : BusSelector  OutputSignals=ABM_NODE.ABM2_MSG.VehLgtAccel
  Bus Selector5 : BusSelector  Commented=on  OutputSignals=vxvRefMs,kapTraj,alpSideSlipAngle,alpSumSlideCurveness,SteerAngleOffset_deg
  Bus Selector8 : BusSelector  Commented=on  OutputSignals=TarLineValid,TarLineC2,TarLineC1,TarLineC0
  Compare To Constant : simulink/Logic and Bit Operations/Compare To Constant  relop=~=  const=0  OutDataTypeStr=boolean
  Compare To Constant1 : simulink/Logic and Bit Operations/Compare To Constant  relop=~=  const=0  OutDataTypeStr=boolean
  Constant : Constant  Value=0
  Constant1 : Constant  Value=3.8  OutDataTypeStr=single
  Constant10 : Constant  Value=0.5  OutDataTypeStr=single
  Constant11 : Constant  Value=57.3  OutDataTypeStr=single
  Constant{2..4,8,12..13} (6 alike) : Constant  Value=0  OutDataTypeStr=uint8
  Constant{5..6,14..15} (4 alike) : Constant  Value=0  OutDataTypeStr=single
  Constant16 : Constant  Value=3
  Constant17 : Constant  Value=2
  Constant18 : Constant  Value=P_HWA_TOS_P0HeadingAngle
  Constant7 : Constant  Value=3.8  OutDataTypeStr=single
  Constant9 : Constant  Value=P_Global_SteeringAngleRatio
  Data Type Conversion{,3,14..15,42,46} (6 alike) : DataTypeConversion  OutDataTypeStr=uint8
  Data Type Conversion{1..2,12..13,16..21,36,41,43..45,48..51} (19 alike) : DataTypeConversion  OutDataTypeStr=single
  Data Type Conversion{4..11,22..35,37..40} (26 alike) : DataTypeConversion
  Data Type Conversion47 : DataTypeConversion  OutDataTypeStr=boolean
  FilterTime3 : Product  Inputs=*//  RndMeth=Zero
  FilterTime6 : Product  Inputs=**  RndMeth=Zero
  Gain9 : Gain  Gain=2
  HWA_Task100ms1 : Subsystem
  ObjMatrixTransit : Subsystem
  Selector : Selector  InputPortWidth=2  IndexOptions=Index vector (dialog)  Indices=1  OutputSizes=1
  Selector{1..12} (12 alike) : Selector  InputPortWidth=20  IndexOptions=Index vector (dialog)  Indices=[1:15]  OutputSizes=1
  Sum1 : Sum  Inputs=|-+
  Sum4 : Sum  Inputs=-+|
  Terminator : Terminator
  VCAN1 : InportShadow  Port=5
  rollingcounter 1 : Subsystem
  ACCP0 : Outport  OutDataTypeStr=Bus: TOS_ACCP0_BUS
  TEM_P0_TARGET_LINE : Outport  Port=2  OutDataTypeStr=Bus: TOS_P0_TARGET_LINE_BUS  PortDimensions=1  BusOutputAsStruct=on
  ACCP2 : Outport  Port=3  OutDataTypeStr=Bus: TOS_ACCP2_BUS
  ACCP3 : Outport  Port=4  OutDataTypeStr=Bus: TOS_ACCP3_BUS
  wires:
  Data Type Conversion51/1 -> HWA_Task100ms1/27(TarLine_A0)
  Data Type Conversion46/1 -> Terminator/1
  Constant18/1 -> Data Type Conversion39/1
  HWA_Task100ms1/46(TargetVyG) -> Data Type Conversion25/1
  Constant17/1 -> Data Type Conversion32/1
  Constant16/1 -> Data Type Conversion29/1
  Selector2/1 -> Bias/1
  [ACCTargetSelectSts] -> Bus Selector6/1
  Bus Selector6/1 -> Compare To Constant1/1, Data Type Conversion42/1  "<P3ID>"
  Data Type Conversion42/1 -> Bus Creator4/1  "IDP3"
  Bus Selector6/2 -> Data Type Conversion43/1  "<P3Dx>"
  Data Type Conversion43/1 -> Add1/1, Bus Creator4/2  "dxP3"
  Bus Selector6/3 -> Data Type Conversion44/1  "<P3Vr>"
  Data Type Conversion44/1 -> Bus Creator4/3  "vxRelP3"
  Bus Selector6/4 -> Data Type Conversion45/1  "<P3ArG>"
  Data Type Conversion45/1 -> Bus Creator4/4  "axAbsGroundP3"
  Add1/1 -> Bus Creator4/5  "rangeP3"
  Constant7/1 -> Add1/2
  Compare To Constant1/1 -> Bus Creator4/6  "targetExistP3"
  Constant8/1 -> Bus Creator4/7  "fu_typeP3"
  Constant12/1 -> Bus Creator4/8  "ObjMovingStateP3"
  Constant13/1 -> Bus Creator4/9  "ObjTypeP3"
  Bus Selector6/5 -> Data Type Conversion48/1  "<P3Dy>"
  Data Type Conversion48/1 -> Bus Creator4/10  "ObjDYP3"
  Constant14/1 -> Bus Creator4/11  "P3CutinProb"
  Constant15/1 -> Bus Creator4/12  "P3HeadingAngle"
  Bus Creator4/1 -> ACCP3/1
  Bus Creator3/1 -> ACCP2/1
  Constant6/1 -> Bus Creator3/12  "P2HeadingAngle"
  Constant5/1 -> Bus Creator3/11  "P2CutinProb"
  Data Type Conversion41/1 -> Bus Creator3/10  "ObjDYP2"
  Bus Selector4/5 -> Data Type Conversion41/1  "<P2Dy>"
  Constant4/1 -> Bus Creator3/9  "ObjTypeP2"
  Constant3/1 -> Bus Creator3/8  "ObjMovingStateP2"
  Constant2/1 -> Bus Creator3/7  "fu_typeP2"
  Compare To Constant/1 -> Bus Creator3/6  "targetExistP2"
  Constant1/1 -> Add/2
  Add/1 -> Bus Creator3/5  "rangeP2"
  Data Type Conversion36/1 -> Bus Creator3/4  "axAbsGroundP2"
  Bus Selector4/4 -> Data Type Conversion36/1  "<P2ArG>"
  Data Type Conversion13/1 -> Bus Creator3/3  "vxRelP2"
  Bus Selector4/3 -> Data Type Conversion13/1  "<P2Vr>"
  Data Type Conversion12/1 -> Bus Creator3/2, Add/1  "dxP2"
  Bus Selector4/2 -> Data Type Conversion12/1  "<P2Dx>"
  Data Type Conversion/1 -> Bus Creator3/1  "IDP2"
  Bus Selector4/1 -> Data Type Conversion/1, Compare To Constant/1  "<P2ID>"
  [ACCTargetSelectSts] -> Bus Selector4/1
  ObjMatrixTransit/1(VisObjSts) -> Bus Selector1/1
  Bus Selector/1 -> ObjMatrixTransit/1(EQ4_OBJ)  "<EQ4_OBJ>"
  Selector12/1 -> HWA_Task100ms1/10(ObjCnt)
  Selector11/1 -> HWA_Task100ms1/12(ObjBrakeLightIndic)
  Selector10/1 -> HWA_Task100ms1/9(ObjWidth_m)
  Selector9/1 -> HWA_Task100ms1/11(ObjMoveSts)
  Selector8/1 -> HWA_Task100ms1/8(ObjArG_ms2)
  Selector7/1 -> HWA_Task100ms1/7(ObjVyG_ms)
  Selector6/1 -> HWA_Task100ms1/6(ObjVxG_ms)
  Selector5/1 -> HWA_Task100ms1/5(ObjClassification)
  Selector4/1 -> HWA_Task100ms1/4(ObjValid)
  Selector3/1 -> HWA_Task100ms1/3(ObjDy_m)
  Bias/1 -> HWA_Task100ms1/2(ObjDx_m)
  Selector1/1 -> HWA_Task100ms1/1(ObjRange_m)
  Selector/1 -> Bus Selector9/1
  Bus Selector/2 -> Selector/1  "<EQ4_LH_ELEM>"
  visMsg/1 -> Bus Selector/1
  Data Type Conversion11/1 -> Bus Creator2/6  "OTL_Range"
  Data Type Conversion10/1 -> Bus Creator2/5  "OTL_C0"
  Data Type Conversion9/1 -> Bus Creator2/4  "OTL_C1"
  Data Type Conversion8/1 -> Bus Creator2/3  "OTL_C2"
  Data Type Conversion7/1 -> Bus Creator2/2  "OTL_C3"
  Data Type Conversion6/1 -> Bus Creator2/1  "OTL_Valid"
  Data Type Conversion5/1 -> Bus Creator2/7  "OTL_Cnt"
  Bus Creator2/1 -> TEM_P0_TARGET_LINE/1
  HWA_Task100ms1/42(bOTL) -> Data Type Conversion8/1  "OTL_C2"
  HWA_Task100ms1/41(aOTL) -> Data Type Conversion7/1  "OTL_C3"
  HWA_Task100ms1/40(OTLValid) -> Data Type Conversion6/1  "OTL_Valid"
  HWA_Task100ms1/43(cOTL) -> Data Type Conversion9/1  "OTL_C1"
  rollingcounter 1/1(cnt) -> Data Type Conversion5/1, Data Type Conversion37/1  "OTL_Cnt"
  HWA_Task100ms1/45(dxMaxOTL) -> Data Type Conversion11/1  "OTL_Range"
  HWA_Task100ms1/44(dOTL) -> Data Type Conversion10/1  "OTL_C0"
  Data Type Conversion4/1 -> Sum1/1
  Bus Selector2/2 -> FilterTime6/2  "<SteerWheelAng>"
  Bus Selector2/1 -> Data Type Conversion4/1  "<SteerWheelAngSign>"
  Sum1/1 -> Gain9/1
  Gain9/1 -> FilterTime6/1
  Constant10/1 -> Sum1/2
  VCAN1/1 -> Bus Selector2/1
  Constant9/1 -> FilterTime3/2
  Bus Selector5/5 -> Sum4/1  "<SteerAngleOffset_deg>"
  FilterTime3/1 -> [alpWheelAngle]
  Sum4/1 -> FilterTime3/1
  Constant11/1 -> FilterTime3/3
  FilterTime6/1 -> Sum4/2
  HWA_Task100ms1/34(aPC0) -> Bus Creator/34
  HWA_Task100ms1/38(bPC1) -> Bus Creator/38
  Bus Selector7/1 -> Data Type Conversion22/1  "<P0ID>"
  Data Type Conversion3/1 -> HWA_Task100ms1/15(Conf)
  Data Type Conversion22/1 -> Bus Creator1/1  "IDP0"
  Data Type Conversion27/1 -> Bus Creator1/6  "rangeP0"
  Data Type Conversion1/1 -> HWA_Task100ms1/13(A2)
  HWA_Task100ms1/2(P2ID) -> Bus Creator/2
  Data Type Conversion2/1 -> HWA_Task100ms1/14(A1)
  Data Type Conversion37/1 -> Bus Creator1/15  "ACCTgtObjCntAlive"
  HWA_Task100ms1/1(P0ID) -> Bus Creator/1
  Bus Selector3/1 -> Data Type Conversion21/1  "<VehLgtAccel>"
  Bus Selector1/9 -> Selector10/1  "<ObjWidth>"
  Data Type Conversion19/1 -> HWA_Task100ms1/21(AlpWheelAngle)
  Bus Selector7/3 -> Data Type Conversion24/1  "<P0Vr>"
  Bus Selector9/1 -> Data Type Conversion1/1  "<LH_Line_First_C2>"
  VIE/1 -> Bus Selector5/1
  Data Type Conversion38/1 -> Bus Creator1/16  "ACCTgtObjExist"
  Bus Selector7/6 -> Data Type Conversion33/1  "<P0Dy>"
  Bus Selector7/2 -> Data Type Conversion23/1  "<P0Dx>"
  Data Type Conversion29/1 -> Bus Creator1/8  "fu_typeP0"
  Bus Selector7/8 -> Data Type Conversion40/1  "<TargetCutIn_b>"
  HWA_Task100ms1/32(ObjqDycHist) -> Bus Creator/32
  Data Type Conversion32/1 -> Bus Creator1/11  "ObjTypeP0"
  Data Type Conversion35/1 -> Bus Creator1/14  "ACCTgtObjAy"
  VCAN/1 -> Bus Selector3/1
  Data Type Conversion34/1 -> Bus Creator1/13  "ACCTgtObjObstcl"
  Bus Selector8/1 -> Data Type Conversion47/1  "<TarLineValid>"
  Bus Selector5/1 -> Data Type Conversion16/1  "<vxvRefMs>"
  Data Type Conversion17/1 -> HWA_Task100ms1/19(kapCurvTraj)
  Data Type Conversion28/1 -> Bus Creator1/7  "targetExistP0"
  Bus Selector1/7 -> Selector7/1  "<ObjLatVel>"
  HWA_Task100ms1/8(P3Vr) -> Bus Creator/8
  Bus Selector1/8 -> Selector8/1  "<ObjLongAccel>"
  Data Type Conversion49/1 -> HWA_Task100ms1/25(TarLine_A2)
  ACCMode/1 -> Data Type Conversion15/1
  HWA_Task100ms1/22(ObjDyc_m) -> Bus Creator/22
  Data Type Conversion18/1 -> HWA_Task100ms1/20(AlpSideSlipAngle)
  Data Type Conversion30/1 -> Bus Creator1/9  "ObjMovingStateP0"
  HWA_Task100ms1/11(P3ArG) -> Bus Creator/11
  Data Type Conversion25/1 -> Bus Creator1/4  "ACCTgtObjVy"
  TimeGap/1 -> Data Type Conversion14/1
  Data Type Conversion23/1 -> Bus Creator1/2  "dxP0"
  Data Type Conversion21/1 -> HWA_Task100ms1/23(LongitudeAcc)
  Bus Creator/1 -> [ACCTargetSelectSts]
  HWA_Task100ms1/31(ObjDycHist) -> Bus Creator/31
  Bus Selector1/5 -> Selector5/1  "<ObjClassification>"
  Bus Selector7/5 -> Data Type Conversion27/1  "<P0Range>"
  Bus Selector5/2 -> Data Type Conversion17/1  "<kapTraj>"
  Bus Selector1/3 -> Selector3/1  "<ObjLatPos>"
  Constant/1 -> Data Type Conversion30/1, Data Type Conversion31/1, Data Type Conversion34/1, Data Type Conversion35/1
  Data Type Conversion47/1 -> HWA_Task100ms1/24(TarLineValid)
  HWA_Task100ms1/4(TargetBrake_b) -> Bus Creator/4
  Data Type Conversion14/1 -> HWA_Task100ms1/16(TimeGap)
  HWA_Task100ms1/15(P0Dy) -> Bus Creator/15
  HWA_Task100ms1/33(dxC0) -> Bus Creator/33
  Data Type Conversion39/1 -> Bus Creator1/17  "P0HeadingAngle"
  HWA_Task100ms1/21(Signal_ACC_TgtObjBarDisp) -> Bus Creator/21
  HWA_Task100ms1/24(ObjVyc_ms) -> Bus Creator/24
  HWA_Task100ms1/16(P2Dy) -> Bus Creator/16
  Bus Selector8/3 -> Data Type Conversion50/1  "<TarLineC1>"
  HWA_Task100ms1/30(ObjPlausRight) -> Bus Creator/30
  HWA_Task100ms1/13(P2Dx) -> Bus Creator/13
  Bus Selector1/11 -> Selector9/1  "<ObjMoveSts>"
  HWA_Task100ms1/35(bPC0) -> Bus Creator/35
  Data Type Conversion16/1 -> HWA_Task100ms1/18(VxvRef_ms)
  Bus Selector9/2 -> Data Type Conversion2/1  "<LH_Line_First_C1>"
  HWA_Task100ms1/18(CutIn_b) -> Bus Creator/18
  HWA_Task100ms1/27(ObjSpwRight) -> Bus Creator/27
  [ACCTargetSelectSts] -> Bus Selector7/1
  HWA_Task100ms1/3(P3ID) -> Bus Creator/3
  HWA_Task100ms1/20(DesireDis) -> Bus Creator/20
  Bus Selector7/4 -> Data Type Conversion26/1  "<P0ArG>"
  Data Type Conversion31/1 -> Bus Creator1/10  "Object_Orientation"
  Data Type Conversion50/1 -> HWA_Task100ms1/26(TarLine_A1)
  Bus Selector1/1 -> Selector1/1  "<ObjRange_m>"
  Bus Selector1/6 -> Selector6/1  "<ObjLongVel>"
  Bus Selector1/12 -> Selector11/1  "<ObjBrakeLightIndic>"
  Bus Selector5/3 -> Data Type Conversion18/1  "<alpSideSlipAngle>"
  HWA_Task100ms1/14(P3Dx) -> Bus Creator/14
  Data Type Conversion33/1 -> Bus Creator1/12  "ObjDYP0"
  Bus Selector5/4 -> Data Type Conversion20/1  "<alpSumSlideCurveness>"
  HWA_Task100ms1/9(P0ArG) -> Bus Creator/9
  HWA_Task100ms1/36(cPC0) -> Bus Creator/36
  HWA_Task100ms1/39(cPC1) -> Bus Creator/39
  HWA_Task100ms1/12(P0Dx) -> Bus Creator/12
  HWA_Task100ms1/17(P3Dy) -> Bus Creator/17
  HWA_Task100ms1/19(TargetExist) -> Bus Creator/19
  Bus Selector1/10 -> Selector12/1  "<ObjCnt>"
  HWA_Task100ms1/10(P2ArG) -> Bus Creator/10
  HWA_Task100ms1/26(ObjSpwLeft) -> Bus Creator/26
  HWA_Task100ms1/37(aPC1) -> Bus Creator/37
  HWA_Task100ms1/5(P0Range) -> Bus Creator/5
  Data Type Conversion26/1 -> Bus Creator1/5  "axAbsGroundP0"
  Bus Selector1/2 -> Selector2/1  "<ObjDx_m>"
  HWA_Task100ms1/28(ObjPlaus) -> Bus Creator/28
  LCKSts/1 -> Data Type Conversion46/1
  Data Type Conversion24/1 -> Bus Creator1/3  "vxRelP0"
  Bus Selector8/2 -> Data Type Conversion49/1  "<TarLineC2>"
  Bus Selector1/4 -> Selector4/1  "<ObjValid>"
  HWA_Task100ms1/7(P2Vr) -> Bus Creator/7
  HWA_Task100ms1/29(ObjPlausLeft) -> Bus Creator/29
  Data Type Conversion40/1 -> Bus Creator1/18  "P0CutInflg"
  desLane/1 -> Bus Selector8/1
  Bus Selector9/3 -> Data Type Conversion3/1  "<LH_Availability_State>"
  [alpWheelAngle] -> Data Type Conversion19/1
  HWA_Task100ms1/25(ObjSpw) -> Bus Creator/25
  HWA_Task100ms1/6(P0Vr) -> Bus Creator/6
  Bus Selector7/7 -> Data Type Conversion38/1, Data Type Conversion28/1  "<TargetExist>"
  Data Type Conversion15/1 -> HWA_Task100ms1/17(ACCMode)
  HWA_Task100ms1/23(ObjVy_ms) -> Bus Creator/23
  Data Type Conversion20/1 -> HWA_Task100ms1/22(alpSumSlideCurveness)
  Bus Selector8/4 -> Data Type Conversion51/1  "<TarLineC0>"
  Bus Creator1/1 -> ACCP0/1

== system Noh_Nofusion/Subsystem3/Subsystem2 ==
  In1 : Inport
  Enable : EnablePort
  Selector : Selector  InputPortWidth=1500  IndexOptions=Index vector (dialog)  Indices=[1:1344]  OutputSizes=1
  Out1 : Outport
  wires:
  In1/1 -> Selector/1
  Selector/1 -> Out1/1

== system Noh_Nofusion/Subsystem4/Simulink Function ==
  fla : TriggerPort  TriggerType=function-call  IsSimulinkFunction=on  FunctionName=fla  FunctionVisibility=scoped  VariantControl=(inherit)
  Constant4 : Constant  Value=P_Global_EQ2RearAxisX_m
  Constant5 : Constant  Value=P_Global_EQ2RearAxisY_m
  MATLAB Function3 : MATLAB Function  TreatAsAtomicUnit=on
  A0 : ArgIn  DisableCoverage=on  OutDataTypeStr=single  ArgumentName=A0
  A1 : ArgIn  DisableCoverage=on  Port=2  OutDataTypeStr=single  ArgumentName=A1
  A2 : ArgIn  DisableCoverage=on  Port=3  OutDataTypeStr=single  ArgumentName=A2
  A3 : ArgIn  DisableCoverage=on  Port=4  OutDataTypeStr=single  ArgumentName=A3
  Range_min : ArgIn  DisableCoverage=on  Port=5  OutDataTypeStr=single  ArgumentName=Range_min
  Range_max : ArgIn  DisableCoverage=on  Port=6  OutDataTypeStr=single  ArgumentName=Range_max
  a0 : ArgOut  DisableCoverage=on  OutDataTypeStr=single  ArgumentName=a0
  a1 : ArgOut  DisableCoverage=on  Port=2  OutDataTypeStr=single  ArgumentName=a1
  a2 : ArgOut  DisableCoverage=on  Port=3  OutDataTypeStr=single  ArgumentName=a2
  a3 : ArgOut  DisableCoverage=on  Port=4  OutDataTypeStr=single  ArgumentName=a3
  Rmin : ArgOut  DisableCoverage=on  Port=5  OutDataTypeStr=single  ArgumentName=Rmin
  Rmax : ArgOut  DisableCoverage=on  Port=6  OutDataTypeStr=single  ArgumentName=Rmax
  wires:
  Constant4/1 -> MATLAB Function3/1(IFV2RearAxis)
  Constant5/1 -> MATLAB Function3/2(IFV2CenterAxis)
  A0/1 -> MATLAB Function3/3(A0)
  A1/1 -> MATLAB Function3/4(A1)
  A2/1 -> MATLAB Function3/5(A2)
  A3/1 -> MATLAB Function3/6(A3)
  Range_min/1 -> MATLAB Function3/7(Range_min)
  Range_max/1 -> MATLAB Function3/8(Range_max)
  MATLAB Function3/1(a0) -> a0/1  "A0"
  MATLAB Function3/2(a1) -> a1/1  "A1"
  MATLAB Function3/3(a2) -> a2/1  "A2"
  MATLAB Function3/4(a3) -> a3/1  "A3"
  MATLAB Function3/5(Rmin) -> Rmin/1  "Rmin"
  MATLAB Function3/6(Rmax) -> Rmax/1  "Rmax"

== system Noh_Nofusion/TOS/Subsystem1 ==
  IfStateMBus : Inport
  IfVIEBus : Inport  Port=2
  IfVCAN : Inport  Port=3  OutDataTypeStr=Bus: VCAN_BUS
  visMsg : Inport  Port=4
  function : TriggerPort  TriggerType=function-call  VariantControl=Variant
  ACCOSM : Subsystem
  Bus Selector16 : BusSelector  OutputSignals=VSM_HMI.LCKSts,VSM_LAT_CTRL
  Bus Selector17 : BusSelector  OutputSignals=VSM_LON_CTRL.ACC_TimeGapSet,VSM_LON_CTRL.ACCSts
  Counter Free-Running : simulink/Sources/Counter Free-Running  NumBits=3  tsamp=-1
  Data Type Conversion : DataTypeConversion
  TOS_ACCP0 : Outport  OutDataTypeStr=Bus: TOS_ACCP0_BUS
  TOS_ACCP1 : Outport  Port=2  OutDataTypeStr=Bus: TOS_ACCP1_BUS  PortDimensions=1  BusOutputAsStruct=on
  ACCP2 : Outport  Port=3  OutDataTypeStr=Bus: TOS_ACCP2_BUS
  ACCP3 : Outport  Port=4  OutDataTypeStr=Bus: TOS_ACCP3_BUS
  TOS_ACCP4 : Outport  Port=5  OutDataTypeStr=Bus: TOS_ACCP4_BUS  PortDimensions=1  BusOutputAsStruct=on
  TOS_ACCP5 : Outport  Port=6  OutDataTypeStr=Bus: TOS_ACCP5_BUS  PortDimensions=1  BusOutputAsStruct=on
  TOS_ELK : Outport  Port=7  OutDataTypeStr=Bus: TOS_ELK_BUS  PortDimensions=1  BusOutputAsStruct=on
  TOS_LCKIE : Outport  Port=8  OutDataTypeStr=Bus: TOS_LCKIE_BUS  PortDimensions=1  BusOutputAsStruct=on
  TOS_AEB_LONOBJ : Outport  Port=9  OutDataTypeStr=Bus: TOS_AEB_LONOBJ_BUS  PortDimensions=1  BusOutputAsStruct=on
  TOS_AEB_LATOBJ : Outport  Port=10  OutDataTypeStr=Bus: TOS_AEB_LATOBJ_BUS  PortDimensions=10  BusOutputAsStruct=on
  TOS_AEB_JAOBJ : Outport  Port=11  OutDataTypeStr=Bus: TOS_AEB_JAOBJ_BUS  PortDimensions=32  BusOutputAsStruct=on
  TOS_P0_TARGET_LINE : Outport  Port=12  OutDataTypeStr=Bus: TOS_P0_TARGET_LINE_BUS
  TOS_UpdateCnt : Outport  Port=13  OutDataTypeStr=uint32  PortDimensions=1  BusOutputAsStruct=on
  wires:
  Data Type Conversion/1 -> TOS_UpdateCnt/1
  Counter Free-Running/1 -> Data Type Conversion/1
  ACCOSM/4(ACCP3) -> ACCP3/1
  ACCOSM/3(ACCP2) -> ACCP2/1
  ACCOSM/2(TEM_P0_TARGET_LINE) -> TOS_P0_TARGET_LINE/1  "TOS_P0_TARGET_LINE"
  ACCOSM/1(ACCP0) -> TOS_ACCP0/1  "TOS_ACCP0"
  IfVCAN/1 -> ACCOSM/5(VCAN)
  Bus Selector17/1 -> ACCOSM/2(TimeGap)  "<ACC_TimeGapSet>"
  Bus Selector17/2 -> ACCOSM/3(ACCMode)  "<ACCSts>"
  Bus Selector16/2 -> ACCOSM/7(desLane)  "<VSM_LAT_CTRL>"
  IfStateMBus/1 -> Bus Selector17/1, Bus Selector16/1
  visMsg/1 -> ACCOSM/1(visMsg)
  Bus Selector16/1 -> ACCOSM/6(LCKSts)  "<LCKSts>"
  IfVIEBus/1 -> ACCOSM/4(VIE)
